simulink library "miniMUTT_rigid_Aero_Lib"  (Simulink 8.4)
settings: Solver=ode45  StartTime=0.0  StopTime=10.0  RelTol=1e-3
values from neighbouring files (symbols this model uses):
  AC = miniMUTT_rigid_config    [UAV_config.m]    (also in UAV_modelconfig.mat = )
libraries: simulink x1
settings Model: Creator=kotik001  LastModifiedBy=pseiler

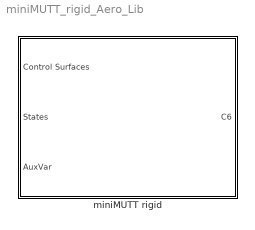
== system miniMUTT_rigid_Aero_Lib ==
  miniMUTT rigid : Subsystem

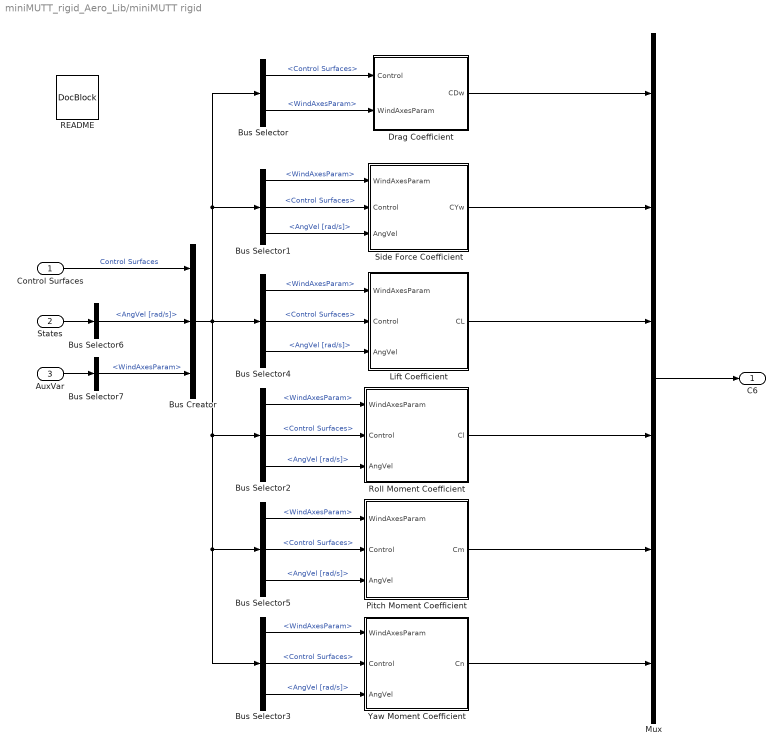
== system miniMUTT_rigid_Aero_Lib/miniMUTT rigid ==
  Control Surfaces : Inport
  States : Inport  Port=2
  AuxVar : Inport  Port=3
  Bus Creator : BusCreator  Inputs=3
  Bus Selector : BusSelector  OutputSignals=Control Surfaces,WindAxesParam
  Bus Selector{1..5} (5 alike) : BusSelector  OutputSignals=WindAxesParam,Control Surfaces,AngVel [rad/s]
  Bus Selector6 : BusSelector  OutputSignals=AngVel [rad/s]
  Bus Selector7 : BusSelector  OutputSignals=WindAxesParam
  Drag Coefficient : Subsystem
  Lift Coefficient : Subsystem
  Mux : Mux  Inputs=6
  Pitch Moment Coefficient : Subsystem
  README : simulink/Model-Wide Utilities/DocBlock  DocumentType=Text
  Roll Moment Coefficient : Subsystem
  Side Force Coefficient : Subsystem
  Yaw Moment Coefficient : Subsystem
  C6 : Outport
  wires:
  Bus Selector/2 -> Drag Coefficient/2(WindAxesParam)  "<WindAxesParam>"
  Bus Selector/1 -> Drag Coefficient/1(Control)  "<Control Surfaces>"
  Bus Selector5/3 -> Pitch Moment Coefficient/3(AngVel)  "<AngVel [rad/s]>"
  Bus Selector5/2 -> Pitch Moment Coefficient/2(Control)  "<Control Surfaces>"
  Bus Selector5/1 -> Pitch Moment Coefficient/1(WindAxesParam)  "<WindAxesParam>"
  Bus Selector4/3 -> Lift Coefficient/3(AngVel)  "<AngVel [rad/s]>"
  Bus Selector4/2 -> Lift Coefficient/2(Control)  "<Control Surfaces>"
  Bus Selector4/1 -> Lift Coefficient/1(WindAxesParam)  "<WindAxesParam>"
  Bus Selector3/3 -> Yaw Moment Coefficient/3(AngVel)  "<AngVel [rad/s]>"
  Bus Selector3/2 -> Yaw Moment Coefficient/2(Control)  "<Control Surfaces>"
  Bus Selector3/1 -> Yaw Moment Coefficient/1(WindAxesParam)  "<WindAxesParam>"
  Bus Selector2/3 -> Roll Moment Coefficient/3(AngVel)  "<AngVel [rad/s]>"
  Bus Selector2/2 -> Roll Moment Coefficient/2(Control)  "<Control Surfaces>"
  Bus Selector2/1 -> Roll Moment Coefficient/1(WindAxesParam)  "<WindAxesParam>"
  Bus Selector1/3 -> Side Force Coefficient/3(AngVel)  "<AngVel [rad/s]>"
  Bus Selector1/2 -> Side Force Coefficient/2(Control)  "<Control Surfaces>"
  Bus Selector1/1 -> Side Force Coefficient/1(WindAxesParam)  "<WindAxesParam>"
  Bus Creator/1 -> Bus Selector1/1, Bus Selector/1, Bus Selector4/1, Bus Selector5/1, Bus Selector3/1, Bus Selector2/1
  Mux/1 -> C6/1
  Yaw Moment Coefficient/1(Cn) -> Mux/6
  Pitch Moment Coefficient/1(Cm) -> Mux/5
  Roll Moment Coefficient/1(Cl) -> Mux/4
  Side Force Coefficient/1(CYw) -> Mux/2
  Drag Coefficient/1(CDw) -> Mux/1
  States/1 -> Bus Selector6/1
  Bus Selector6/1 -> Bus Creator/2  "<AngVel [rad/s]>"
  Lift Coefficient/1(CL) -> Mux/3
  AuxVar/1 -> Bus Selector7/1
  Bus Selector7/1 -> Bus Creator/3  "<WindAxesParam>"
  Control Surfaces/1 -> Bus Creator/1  "Control Surfaces"

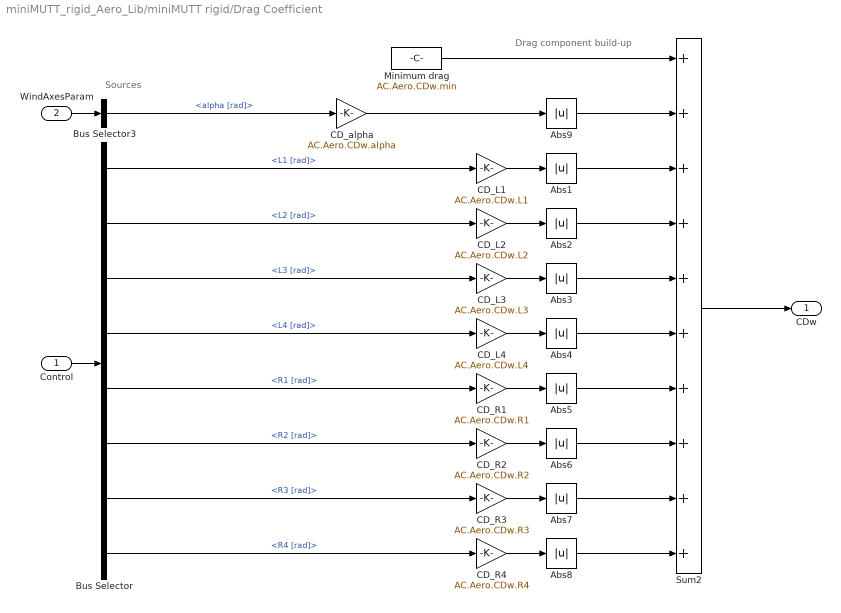
== system miniMUTT_rigid_Aero_Lib/miniMUTT rigid/Drag Coefficient ==
  note: Sources
  note: Drag component build-up
  Control : Inport
  WindAxesParam : Inport  Port=2
  Abs{1..9} (9 alike) : Abs  SaturateOnIntegerOverflow=on
  Bus Selector : BusSelector  OutputSignals=L1 [rad],L2 [rad],L3 [rad],L4 [rad],R1 [rad],R2 [rad],R3 [rad],R4 [rad]
  Bus Selector3 : BusSelector  OutputSignals=alpha [rad]
  CD_L1 : Gain  Gain=AC.Aero.CDw.L1  SaturateOnIntegerOverflow=on  OutDataTypeStr=Inherit: Same as input  ParamDataTypeStr=Inherit: Same as input
  CD_L2 : Gain  Gain=AC.Aero.CDw.L2  SaturateOnIntegerOverflow=on  OutDataTypeStr=Inherit: Same as input  ParamDataTypeStr=Inherit: Same as input
  CD_L3 : Gain  Gain=AC.Aero.CDw.L3  SaturateOnIntegerOverflow=on  OutDataTypeStr=Inherit: Same as input  ParamDataTypeStr=Inherit: Same as input
  CD_L4 : Gain  Gain=AC.Aero.CDw.L4  SaturateOnIntegerOverflow=on  OutDataTypeStr=Inherit: Same as input  ParamDataTypeStr=Inherit: Same as input
  CD_R1 : Gain  Gain=AC.Aero.CDw.R1  SaturateOnIntegerOverflow=on  OutDataTypeStr=Inherit: Same as input  ParamDataTypeStr=Inherit: Same as input
  CD_R2 : Gain  Gain=AC.Aero.CDw.R2  SaturateOnIntegerOverflow=on  OutDataTypeStr=Inherit: Same as input  ParamDataTypeStr=Inherit: Same as input
  CD_R3 : Gain  Gain=AC.Aero.CDw.R3  SaturateOnIntegerOverflow=on  OutDataTypeStr=Inherit: Same as input  ParamDataTypeStr=Inherit: Same as input
  CD_R4 : Gain  Gain=AC.Aero.CDw.R4  SaturateOnIntegerOverflow=on  OutDataTypeStr=Inherit: Same as input  ParamDataTypeStr=Inherit: Same as input
  CD_alpha : Gain  Gain=AC.Aero.CDw.alpha  SaturateOnIntegerOverflow=on  OutDataTypeStr=Inherit: Same as input  ParamDataTypeStr=Inherit: Same as input
  Minimum drag : Constant  Value=AC.Aero.CDw.min
  Sum2 : Sum  Inputs=++++++++++  SaturateOnIntegerOverflow=on  InputSameDT=on  OutDataTypeStr=Inherit: Same as first input
  CDw : Outport
  wires:
  WindAxesParam/1 -> Bus Selector3/1
  Bus Selector3/1 -> CD_alpha/1  "<alpha [rad]>"
  Bus Selector/7 -> CD_R3/1  "<R3 [rad]>"
  CD_R3/1 -> Abs7/1
  CD_R4/1 -> Abs8/1
  Abs8/1 -> Sum2/10
  Abs7/1 -> Sum2/9
  Bus Selector/8 -> CD_R4/1  "<R4 [rad]>"
  Bus Selector/5 -> CD_R1/1  "<R1 [rad]>"
  Bus Selector/1 -> CD_L1/1  "<L1 [rad]>"
  Bus Selector/2 -> CD_L2/1  "<L2 [rad]>"
  Control/1 -> Bus Selector/1
  Minimum drag/1 -> Sum2/1
  CD_R1/1 -> Abs5/1
  CD_L1/1 -> Abs1/1
  CD_L4/1 -> Abs4/1
  CD_L2/1 -> Abs2/1
  Sum2/1 -> CDw/1
  Abs1/1 -> Sum2/3
  Abs2/1 -> Sum2/4
  Bus Selector/4 -> CD_L4/1  "<L4 [rad]>"
  Abs4/1 -> Sum2/6
  CD_L3/1 -> Abs3/1
  Abs3/1 -> Sum2/5
  Bus Selector/3 -> CD_L3/1  "<L3 [rad]>"
  CD_R2/1 -> Abs6/1
  Abs6/1 -> Sum2/8
  Abs5/1 -> Sum2/7
  Bus Selector/6 -> CD_R2/1  "<R2 [rad]>"
  Abs9/1 -> Sum2/2
  CD_alpha/1 -> Abs9/1

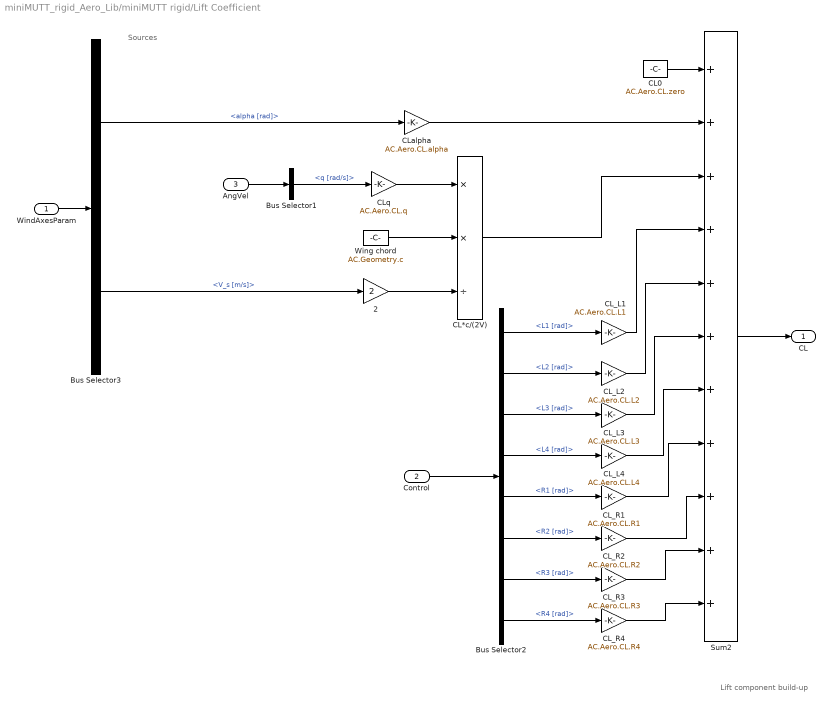
== system miniMUTT_rigid_Aero_Lib/miniMUTT rigid/Lift Coefficient ==
  note: Sources
  note: Lift component build-up
  WindAxesParam : Inport
  Control : Inport  Port=2
  AngVel : Inport  Port=3
  2 : Gain  Gain=2  SaturateOnIntegerOverflow=on  OutDataTypeStr=Inherit: Same as input  ParamDataTypeStr=Inherit: Same as input
  Bus Selector1 : BusSelector  OutputSignals=q [rad/s]
  Bus Selector2 : BusSelector  OutputSignals=L1 [rad],L2 [rad],L3 [rad],L4 [rad],R1 [rad],R2 [rad],R3 [rad],R4 [rad]
  Bus Selector3 : BusSelector  OutputSignals=alpha [rad],V_s [m/s]
  CL*c/(2V) : Product  Inputs=**/  SaturateOnIntegerOverflow=on  InputSameDT=on  OutDataTypeStr=Inherit: Same as first input
  CL0 : Constant  Value=AC.Aero.CL.zero
  CL_L1 : Gain  Gain=AC.Aero.CL.L1  SaturateOnIntegerOverflow=on  OutDataTypeStr=Inherit: Same as input  ParamDataTypeStr=Inherit: Same as input
  CL_L2 : Gain  Gain=AC.Aero.CL.L2  SaturateOnIntegerOverflow=on  OutDataTypeStr=Inherit: Same as input  ParamDataTypeStr=Inherit: Same as input
  CL_L3 : Gain  Gain=AC.Aero.CL.L3  SaturateOnIntegerOverflow=on  OutDataTypeStr=Inherit: Same as input  ParamDataTypeStr=Inherit: Same as input
  CL_L4 : Gain  Gain=AC.Aero.CL.L4  SaturateOnIntegerOverflow=on  OutDataTypeStr=Inherit: Same as input  ParamDataTypeStr=Inherit: Same as input
  CL_R1 : Gain  Gain=AC.Aero.CL.R1  SaturateOnIntegerOverflow=on  OutDataTypeStr=Inherit: Same as input  ParamDataTypeStr=Inherit: Same as input
  CL_R2 : Gain  Gain=AC.Aero.CL.R2  SaturateOnIntegerOverflow=on  OutDataTypeStr=Inherit: Same as input  ParamDataTypeStr=Inherit: Same as input
  CL_R3 : Gain  Gain=AC.Aero.CL.R3  SaturateOnIntegerOverflow=on  OutDataTypeStr=Inherit: Same as input  ParamDataTypeStr=Inherit: Same as input
  CL_R4 : Gain  Gain=AC.Aero.CL.R4  SaturateOnIntegerOverflow=on  OutDataTypeStr=Inherit: Same as input  ParamDataTypeStr=Inherit: Same as input
  CLalpha : Gain  Gain=AC.Aero.CL.alpha  SaturateOnIntegerOverflow=on  OutDataTypeStr=Inherit: Same as input  ParamDataTypeStr=Inherit: Same as input
  CLq : Gain  Gain=AC.Aero.CL.q  SaturateOnIntegerOverflow=on  OutDataTypeStr=Inherit: Same as input  ParamDataTypeStr=Inherit: Same as input
  Sum2 : Sum  Inputs=+++++++++++  SaturateOnIntegerOverflow=on  InputSameDT=on  OutDataTypeStr=Inherit: Same as first input
  Wing chord : Constant  Value=AC.Geometry.c
  CL : Outport
  wires:
  CL_R4/1 -> Sum2/11
  CL_R3/1 -> Sum2/10
  CL_R2/1 -> Sum2/9
  Bus Selector2/6 -> CL_R2/1  "<R2 [rad]>"
  Bus Selector2/7 -> CL_R3/1  "<R3 [rad]>"
  Bus Selector2/8 -> CL_R4/1  "<R4 [rad]>"
  WindAxesParam/1 -> Bus Selector3/1
  CL0/1 -> Sum2/1
  CLalpha/1 -> Sum2/2
  Sum2/1 -> CL/1
  Bus Selector3/1 -> CLalpha/1  "<alpha [rad]>"
  Control/1 -> Bus Selector2/1
  Bus Selector2/1 -> CL_L1/1  "<L1 [rad]>"
  2/1 -> CL*c/(2V)/3
  Wing chord/1 -> CL*c/(2V)/2
  CLq/1 -> CL*c/(2V)/1
  AngVel/1 -> Bus Selector1/1
  Bus Selector1/1 -> CLq/1  "<q [rad/s]>"
  Bus Selector3/2 -> 2/1  "<V_s [m/s]>"
  CL*c/(2V)/1 -> Sum2/3
  CL_L1/1 -> Sum2/4
  Bus Selector2/2 -> CL_L2/1  "<L2 [rad]>"
  Bus Selector2/3 -> CL_L3/1  "<L3 [rad]>"
  Bus Selector2/4 -> CL_L4/1  "<L4 [rad]>"
  Bus Selector2/5 -> CL_R1/1  "<R1 [rad]>"
  CL_L4/1 -> Sum2/7
  CL_R1/1 -> Sum2/8
  CL_L3/1 -> Sum2/6
  CL_L2/1 -> Sum2/5

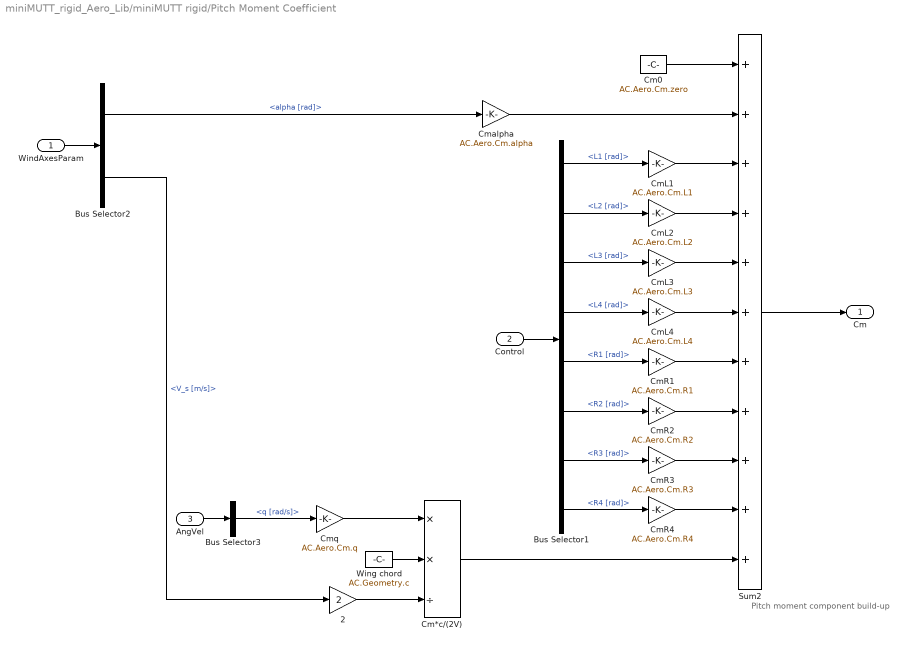
== system miniMUTT_rigid_Aero_Lib/miniMUTT rigid/Pitch Moment Coefficient ==
  note: Pitch moment component build-up
  WindAxesParam : Inport
  Control : Inport  Port=2
  AngVel : Inport  Port=3
  2 : Gain  Gain=2  SaturateOnIntegerOverflow=on  OutDataTypeStr=Inherit: Same as input  ParamDataTypeStr=Inherit: Same as input
  Bus Selector1 : BusSelector  OutputSignals=L1 [rad],L2 [rad],L3 [rad],L4 [rad],R1 [rad],R2 [rad],R3 [rad],R4 [rad]
  Bus Selector2 : BusSelector  OutputSignals=alpha [rad],V_s [m/s]
  Bus Selector3 : BusSelector  OutputSignals=q [rad/s]
  Cm*c/(2V) : Product  Inputs=**/  SaturateOnIntegerOverflow=on  RndMeth=Zero  InputSameDT=on  OutDataTypeStr=Inherit: Same as first input
  Cm0 : Constant  Value=AC.Aero.Cm.zero
  CmL1 : Gain  Gain=AC.Aero.Cm.L1  SaturateOnIntegerOverflow=on  OutDataTypeStr=Inherit: Same as input  ParamDataTypeStr=Inherit: Same as input
  CmL2 : Gain  Gain=AC.Aero.Cm.L2  SaturateOnIntegerOverflow=on  OutDataTypeStr=Inherit: Same as input  ParamDataTypeStr=Inherit: Same as input
  CmL3 : Gain  Gain=AC.Aero.Cm.L3  SaturateOnIntegerOverflow=on  OutDataTypeStr=Inherit: Same as input  ParamDataTypeStr=Inherit: Same as input
  CmL4 : Gain  Gain=AC.Aero.Cm.L4  SaturateOnIntegerOverflow=on  OutDataTypeStr=Inherit: Same as input  ParamDataTypeStr=Inherit: Same as input
  CmR1 : Gain  Gain=AC.Aero.Cm.R1  SaturateOnIntegerOverflow=on  OutDataTypeStr=Inherit: Same as input  ParamDataTypeStr=Inherit: Same as input
  CmR2 : Gain  Gain=AC.Aero.Cm.R2  SaturateOnIntegerOverflow=on  OutDataTypeStr=Inherit: Same as input  ParamDataTypeStr=Inherit: Same as input
  CmR3 : Gain  Gain=AC.Aero.Cm.R3  SaturateOnIntegerOverflow=on  OutDataTypeStr=Inherit: Same as input  ParamDataTypeStr=Inherit: Same as input
  CmR4 : Gain  Gain=AC.Aero.Cm.R4  SaturateOnIntegerOverflow=on  OutDataTypeStr=Inherit: Same as input  ParamDataTypeStr=Inherit: Same as input
  Cmalpha : Gain  Gain=AC.Aero.Cm.alpha  SaturateOnIntegerOverflow=on  OutDataTypeStr=Inherit: Same as input  ParamDataTypeStr=Inherit: Same as input
  Cmq : Gain  Gain=AC.Aero.Cm.q  SaturateOnIntegerOverflow=on  OutDataTypeStr=Inherit: Same as input  ParamDataTypeStr=Inherit: Same as input
  Sum2 : Sum  Inputs=+++++++++++  SaturateOnIntegerOverflow=on  InputSameDT=on  OutDataTypeStr=Inherit: Same as first input
  Wing chord : Constant  Value=AC.Geometry.c
  Cm : Outport
  wires:
  CmR2/1 -> Sum2/8
  CmR3/1 -> Sum2/9
  CmR4/1 -> Sum2/10
  Bus Selector1/6 -> CmR2/1  "<R2 [rad]>"
  Bus Selector1/7 -> CmR3/1  "<R3 [rad]>"
  Bus Selector1/8 -> CmR4/1  "<R4 [rad]>"
  Cm*c/(2V)/1 -> Sum2/11
  WindAxesParam/1 -> Bus Selector2/1
  Control/1 -> Bus Selector1/1
  AngVel/1 -> Bus Selector3/1
  2/1 -> Cm*c/(2V)/3
  Wing chord/1 -> Cm*c/(2V)/2
  Cmq/1 -> Cm*c/(2V)/1
  Cm0/1 -> Sum2/1
  Cmalpha/1 -> Sum2/2
  Sum2/1 -> Cm/1
  Bus Selector3/1 -> Cmq/1  "<q [rad/s]>"
  Bus Selector2/1 -> Cmalpha/1  "<alpha [rad]>"
  Bus Selector2/2 -> 2/1  "<V_s [m/s]>"
  CmL1/1 -> Sum2/3
  CmL2/1 -> Sum2/4
  CmL3/1 -> Sum2/5
  CmL4/1 -> Sum2/6
  CmR1/1 -> Sum2/7
  Bus Selector1/1 -> CmL1/1  "<L1 [rad]>"
  Bus Selector1/2 -> CmL2/1  "<L2 [rad]>"
  Bus Selector1/3 -> CmL3/1  "<L3 [rad]>"
  Bus Selector1/4 -> CmL4/1  "<L4 [rad]>"
  Bus Selector1/5 -> CmR1/1  "<R1 [rad]>"

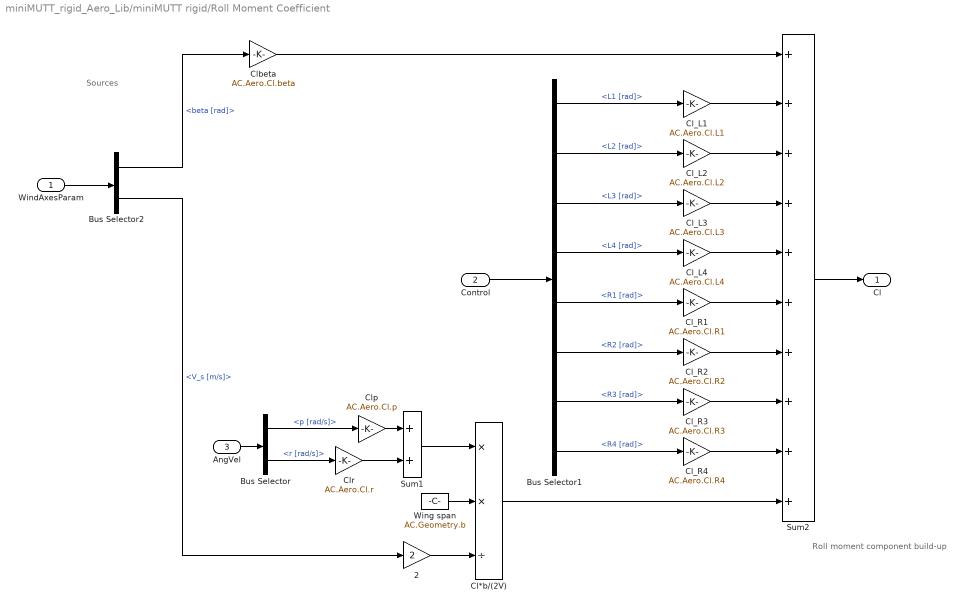
== system miniMUTT_rigid_Aero_Lib/miniMUTT rigid/Roll Moment Coefficient ==
  note: Sources
  note: Roll moment component build-up
  WindAxesParam : Inport
  Control : Inport  Port=2
  AngVel : Inport  Port=3
  2 : Gain  Gain=2  SaturateOnIntegerOverflow=on  OutDataTypeStr=Inherit: Same as input  ParamDataTypeStr=Inherit: Same as input
  Bus Selector : BusSelector  OutputSignals=p [rad/s],r [rad/s]
  Bus Selector1 : BusSelector  OutputSignals=L1 [rad],L2 [rad],L3 [rad],L4 [rad],R1 [rad],R2 [rad],R3 [rad],R4 [rad]
  Bus Selector2 : BusSelector  OutputSignals=beta [rad],V_s [m/s]
  Cl*b/(2V) : Product  Inputs=**/  SaturateOnIntegerOverflow=on  RndMeth=Zero  InputSameDT=on  OutDataTypeStr=Inherit: Same as first input
  Cl_L1 : Gain  Gain=AC.Aero.Cl.L1  SaturateOnIntegerOverflow=on  OutDataTypeStr=Inherit: Same as input  ParamDataTypeStr=Inherit: Same as input
  Cl_L2 : Gain  Gain=AC.Aero.Cl.L2  SaturateOnIntegerOverflow=on  OutDataTypeStr=Inherit: Same as input  ParamDataTypeStr=Inherit: Same as input
  Cl_L3 : Gain  Gain=AC.Aero.Cl.L3  SaturateOnIntegerOverflow=on  OutDataTypeStr=Inherit: Same as input  ParamDataTypeStr=Inherit: Same as input
  Cl_L4 : Gain  Gain=AC.Aero.Cl.L4  SaturateOnIntegerOverflow=on  OutDataTypeStr=Inherit: Same as input  ParamDataTypeStr=Inherit: Same as input
  Cl_R1 : Gain  Gain=AC.Aero.Cl.R1  SaturateOnIntegerOverflow=on  OutDataTypeStr=Inherit: Same as input  ParamDataTypeStr=Inherit: Same as input
  Cl_R2 : Gain  Gain=AC.Aero.Cl.R2  SaturateOnIntegerOverflow=on  OutDataTypeStr=Inherit: Same as input  ParamDataTypeStr=Inherit: Same as input
  Cl_R3 : Gain  Gain=AC.Aero.Cl.R3  SaturateOnIntegerOverflow=on  OutDataTypeStr=Inherit: Same as input  ParamDataTypeStr=Inherit: Same as input
  Cl_R4 : Gain  Gain=AC.Aero.Cl.R4  SaturateOnIntegerOverflow=on  OutDataTypeStr=Inherit: Same as input  ParamDataTypeStr=Inherit: Same as input
  Clbeta : Gain  Gain=AC.Aero.Cl.beta  SaturateOnIntegerOverflow=on  OutDataTypeStr=Inherit: Same as input  ParamDataTypeStr=Inherit: Same as input
  Clp : Gain  Gain=AC.Aero.Cl.p  SaturateOnIntegerOverflow=on  OutDataTypeStr=Inherit: Same as input  ParamDataTypeStr=Inherit: Same as input
  Clr : Gain  Gain=AC.Aero.Cl.r  SaturateOnIntegerOverflow=on  OutDataTypeStr=Inherit: Same as input  ParamDataTypeStr=Inherit: Same as input
  Sum1 : Sum  SaturateOnIntegerOverflow=on  InputSameDT=on  OutDataTypeStr=Inherit: Same as first input
  Sum2 : Sum  Inputs=++++++++++  SaturateOnIntegerOverflow=on  InputSameDT=on  OutDataTypeStr=Inherit: Same as first input
  Wing span : Constant  Value=AC.Geometry.b
  Cl : Outport
  wires:
  Control/1 -> Bus Selector1/1
  Bus Selector1/6 -> Cl_R2/1  "<R2 [rad]>"
  Cl_R2/1 -> Sum2/7
  Bus Selector1/7 -> Cl_R3/1  "<R3 [rad]>"
  Bus Selector1/8 -> Cl_R4/1  "<R4 [rad]>"
  Cl_R3/1 -> Sum2/8
  Cl_R4/1 -> Sum2/9
  Cl*b/(2V)/1 -> Sum2/10
  Clp/1 -> Sum1/1
  Clr/1 -> Sum1/2
  Sum1/1 -> Cl*b/(2V)/1
  Wing span/1 -> Cl*b/(2V)/2
  2/1 -> Cl*b/(2V)/3
  WindAxesParam/1 -> Bus Selector2/1
  AngVel/1 -> Bus Selector/1
  Clbeta/1 -> Sum2/1
  Sum2/1 -> Cl/1
  Bus Selector/1 -> Clp/1  "<p [rad/s]>"
  Bus Selector/2 -> Clr/1  "<r [rad/s]>"
  Bus Selector1/1 -> Cl_L1/1  "<L1 [rad]>"
  Bus Selector2/1 -> Clbeta/1  "<beta [rad]>"
  Bus Selector2/2 -> 2/1  "<V_s [m/s]>"
  Cl_L1/1 -> Sum2/2
  Cl_L2/1 -> Sum2/3
  Bus Selector1/2 -> Cl_L2/1  "<L2 [rad]>"
  Bus Selector1/3 -> Cl_L3/1  "<L3 [rad]>"
  Cl_L3/1 -> Sum2/4
  Bus Selector1/4 -> Cl_L4/1  "<L4 [rad]>"
  Bus Selector1/5 -> Cl_R1/1  "<R1 [rad]>"
  Cl_L4/1 -> Sum2/5
  Cl_R1/1 -> Sum2/6

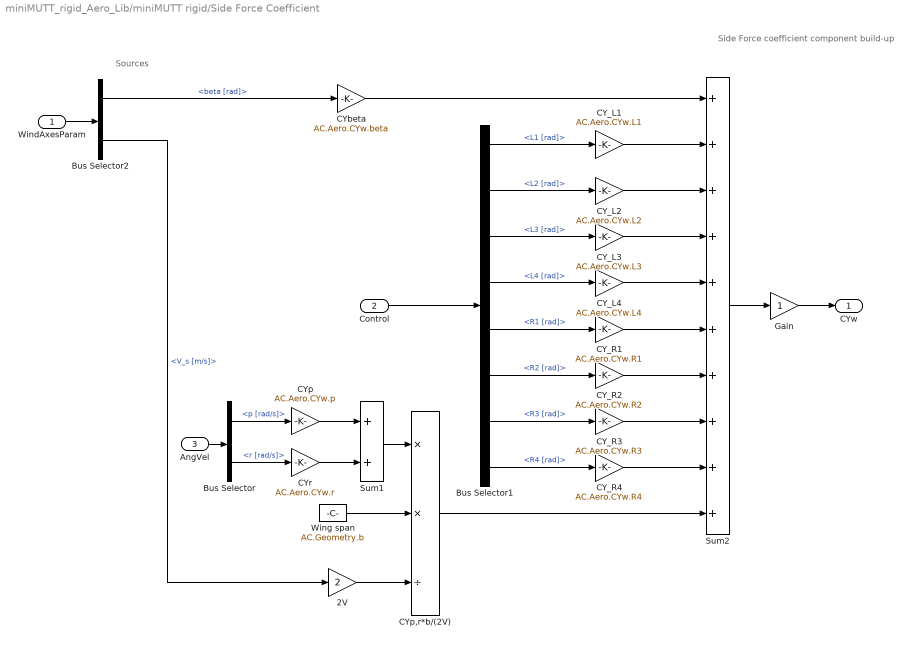
== system miniMUTT_rigid_Aero_Lib/miniMUTT rigid/Side Force Coefficient ==
  note: Sources
  note: Side Force coefficient component build-up
  WindAxesParam : Inport
  Control : Inport  Port=2
  AngVel : Inport  Port=3
  2V : Gain  Gain=2  SaturateOnIntegerOverflow=on  OutDataTypeStr=Inherit: Same as input  ParamDataTypeStr=Inherit: Same as input
  Bus Selector : BusSelector  OutputSignals=p [rad/s],r [rad/s]
  Bus Selector1 : BusSelector  OutputSignals=L1 [rad],L2 [rad],L3 [rad],L4 [rad],R1 [rad],R2 [rad],R3 [rad],R4 [rad]
  Bus Selector2 : BusSelector  OutputSignals=beta [rad],V_s [m/s]
  CY_L1 : Gain  Gain=AC.Aero.CYw.L1  SaturateOnIntegerOverflow=on  OutDataTypeStr=Inherit: Same as input  ParamDataTypeStr=Inherit: Same as input
  CY_L2 : Gain  Gain=AC.Aero.CYw.L2  SaturateOnIntegerOverflow=on  OutDataTypeStr=Inherit: Same as input  ParamDataTypeStr=Inherit: Same as input
  CY_L3 : Gain  Gain=AC.Aero.CYw.L3  SaturateOnIntegerOverflow=on  OutDataTypeStr=Inherit: Same as input  ParamDataTypeStr=Inherit: Same as input
  CY_L4 : Gain  Gain=AC.Aero.CYw.L4  SaturateOnIntegerOverflow=on  OutDataTypeStr=Inherit: Same as input  ParamDataTypeStr=Inherit: Same as input
  CY_R1 : Gain  Gain=AC.Aero.CYw.R1  SaturateOnIntegerOverflow=on  OutDataTypeStr=Inherit: Same as input  ParamDataTypeStr=Inherit: Same as input
  CY_R2 : Gain  Gain=AC.Aero.CYw.R2  SaturateOnIntegerOverflow=on  OutDataTypeStr=Inherit: Same as input  ParamDataTypeStr=Inherit: Same as input
  CY_R3 : Gain  Gain=AC.Aero.CYw.R3  SaturateOnIntegerOverflow=on  OutDataTypeStr=Inherit: Same as input  ParamDataTypeStr=Inherit: Same as input
  CY_R4 : Gain  Gain=AC.Aero.CYw.R4  SaturateOnIntegerOverflow=on  OutDataTypeStr=Inherit: Same as input  ParamDataTypeStr=Inherit: Same as input
  CYbeta : Gain  Gain=AC.Aero.CYw.beta  SaturateOnIntegerOverflow=on  OutDataTypeStr=Inherit: Same as input  ParamDataTypeStr=Inherit: Same as input
  CYp : Gain  Gain=AC.Aero.CYw.p  SaturateOnIntegerOverflow=on  OutDataTypeStr=Inherit: Same as input  ParamDataTypeStr=Inherit: Same as input
  CYp,r*b/(2V) : Product  Inputs=**/  SaturateOnIntegerOverflow=on  RndMeth=Zero  InputSameDT=on  OutDataTypeStr=Inherit: Same as first input
  CYr : Gain  Gain=AC.Aero.CYw.r  SaturateOnIntegerOverflow=on  OutDataTypeStr=Inherit: Same as input  ParamDataTypeStr=Inherit: Same as input
  Gain : Gain
  Sum1 : Sum  SaturateOnIntegerOverflow=on  InputSameDT=on  OutDataTypeStr=Inherit: Same as first input
  Sum2 : Sum  Inputs=++++++++++  SaturateOnIntegerOverflow=on  InputSameDT=on  OutDataTypeStr=Inherit: Same as first input
  Wing span : Constant  Value=AC.Geometry.b
  CYw : Outport
  wires:
  CY_R4/1 -> Sum2/9
  CY_R3/1 -> Sum2/8
  Bus Selector1/8 -> CY_R4/1  "<R4 [rad]>"
  Bus Selector1/7 -> CY_R3/1  "<R3 [rad]>"
  CY_R2/1 -> Sum2/7
  CY_R1/1 -> Sum2/6
  CY_L4/1 -> Sum2/5
  Bus Selector1/4 -> CY_L4/1  "<L4 [rad]>"
  Bus Selector1/6 -> CY_R2/1  "<R2 [rad]>"
  Bus Selector1/5 -> CY_R1/1  "<R1 [rad]>"
  CYp,r*b/(2V)/1 -> Sum2/10
  CYp/1 -> Sum1/1
  CYr/1 -> Sum1/2
  Sum1/1 -> CYp,r*b/(2V)/1
  Wing span/1 -> CYp,r*b/(2V)/2
  2V/1 -> CYp,r*b/(2V)/3
  WindAxesParam/1 -> Bus Selector2/1
  Bus Selector/1 -> CYp/1  "<p [rad/s]>"
  CYbeta/1 -> Sum2/1
  CY_L1/1 -> Sum2/2
  Sum2/1 -> Gain/1
  AngVel/1 -> Bus Selector/1
  Bus Selector/2 -> CYr/1  "<r [rad/s]>"
  Control/1 -> Bus Selector1/1
  Bus Selector1/1 -> CY_L1/1  "<L1 [rad]>"
  Bus Selector1/3 -> CY_L3/1  "<L3 [rad]>"
  Bus Selector2/2 -> 2V/1  "<V_s [m/s]>"
  Bus Selector2/1 -> CYbeta/1  "<beta [rad]>"
  Gain/1 -> CYw/1
  CY_L3/1 -> Sum2/4
  Bus Selector1/2 -> CY_L2/1  "<L2 [rad]>"
  CY_L2/1 -> Sum2/3

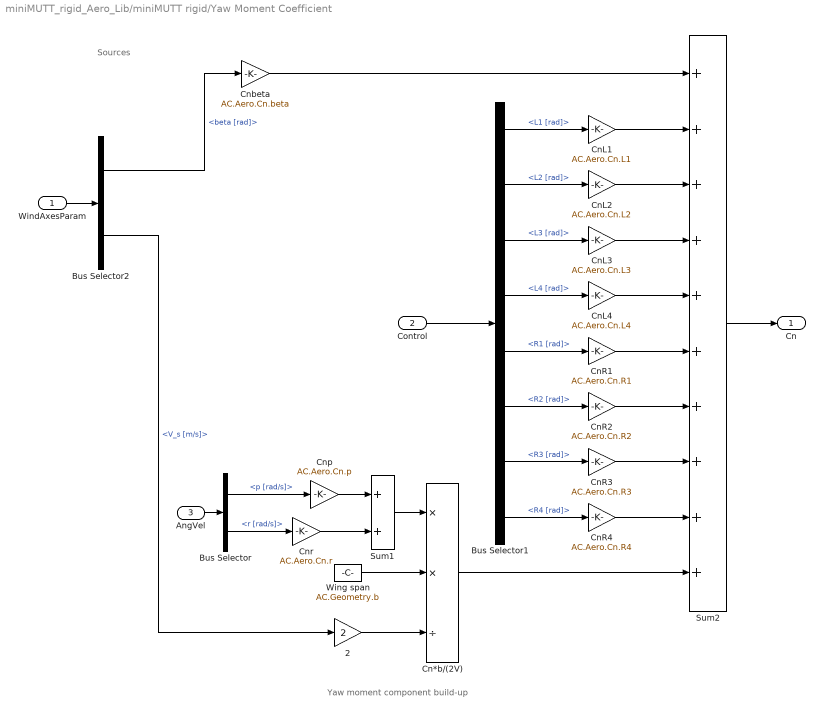
== system miniMUTT_rigid_Aero_Lib/miniMUTT rigid/Yaw Moment Coefficient ==
  note: Yaw moment component build-up
  note: Sources
  WindAxesParam : Inport
  Control : Inport  Port=2
  AngVel : Inport  Port=3
  2 : Gain  Gain=2  SaturateOnIntegerOverflow=on  OutDataTypeStr=Inherit: Same as input  ParamDataTypeStr=Inherit: Same as input
  Bus Selector : BusSelector  OutputSignals=p [rad/s],r [rad/s]
  Bus Selector1 : BusSelector  OutputSignals=L1 [rad],L2 [rad],L3 [rad],L4 [rad],R1 [rad],R2 [rad],R3 [rad],R4 [rad]
  Bus Selector2 : BusSelector  OutputSignals=beta [rad],V_s [m/s]
  Cn*b/(2V) : Product  Inputs=**/  SaturateOnIntegerOverflow=on  RndMeth=Zero  InputSameDT=on  OutDataTypeStr=Inherit: Same as first input
  CnL1 : Gain  Gain=AC.Aero.Cn.L1  SaturateOnIntegerOverflow=on  OutDataTypeStr=Inherit: Same as input  ParamDataTypeStr=Inherit: Same as input
  CnL2 : Gain  Gain=AC.Aero.Cn.L2  SaturateOnIntegerOverflow=on  OutDataTypeStr=Inherit: Same as input  ParamDataTypeStr=Inherit: Same as input
  CnL3 : Gain  Gain=AC.Aero.Cn.L3  SaturateOnIntegerOverflow=on  OutDataTypeStr=Inherit: Same as input  ParamDataTypeStr=Inherit: Same as input
  CnL4 : Gain  Gain=AC.Aero.Cn.L4  SaturateOnIntegerOverflow=on  OutDataTypeStr=Inherit: Same as input  ParamDataTypeStr=Inherit: Same as input
  CnR1 : Gain  Gain=AC.Aero.Cn.R1  SaturateOnIntegerOverflow=on  OutDataTypeStr=Inherit: Same as input  ParamDataTypeStr=Inherit: Same as input
  CnR2 : Gain  Gain=AC.Aero.Cn.R2  SaturateOnIntegerOverflow=on  OutDataTypeStr=Inherit: Same as input  ParamDataTypeStr=Inherit: Same as input
  CnR3 : Gain  Gain=AC.Aero.Cn.R3  SaturateOnIntegerOverflow=on  OutDataTypeStr=Inherit: Same as input  ParamDataTypeStr=Inherit: Same as input
  CnR4 : Gain  Gain=AC.Aero.Cn.R4  SaturateOnIntegerOverflow=on  OutDataTypeStr=Inherit: Same as input  ParamDataTypeStr=Inherit: Same as input
  Cnbeta : Gain  Gain=AC.Aero.Cn.beta  SaturateOnIntegerOverflow=on  OutDataTypeStr=Inherit: Same as input  ParamDataTypeStr=Inherit: Same as input
  Cnp : Gain  Gain=AC.Aero.Cn.p  SaturateOnIntegerOverflow=on  OutDataTypeStr=Inherit: Same as input  ParamDataTypeStr=Inherit: Same as input
  Cnr : Gain  Gain=AC.Aero.Cn.r  SaturateOnIntegerOverflow=on  OutDataTypeStr=Inherit: Same as input  ParamDataTypeStr=Inherit: Same as input
  Sum1 : Sum  SaturateOnIntegerOverflow=on  InputSameDT=on  OutDataTypeStr=Inherit: Same as first input
  Sum2 : Sum  Inputs=++++++++++  SaturateOnIntegerOverflow=on  InputSameDT=on  OutDataTypeStr=Inherit: Same as first input
  Wing span : Constant  Value=AC.Geometry.b
  Cn : Outport
  wires:
  CnR2/1 -> Sum2/7
  CnR3/1 -> Sum2/8
  CnR4/1 -> Sum2/9
  Bus Selector1/6 -> CnR2/1  "<R2 [rad]>"
  Bus Selector1/7 -> CnR3/1  "<R3 [rad]>"
  Bus Selector1/8 -> CnR4/1  "<R4 [rad]>"
  Cn*b/(2V)/1 -> Sum2/10
  Sum2/1 -> Cn/1
  Cnbeta/1 -> Sum2/1
  AngVel/1 -> Bus Selector/1
  WindAxesParam/1 -> Bus Selector2/1
  2/1 -> Cn*b/(2V)/3
  Wing span/1 -> Cn*b/(2V)/2
  Sum1/1 -> Cn*b/(2V)/1
  Cnr/1 -> Sum1/2
  Cnp/1 -> Sum1/1
  Bus Selector/1 -> Cnp/1  "<p [rad/s]>"
  Bus Selector/2 -> Cnr/1  "<r [rad/s]>"
  Control/1 -> Bus Selector1/1
  Bus Selector2/1 -> Cnbeta/1  "<beta [rad]>"
  Bus Selector2/2 -> 2/1  "<V_s [m/s]>"
  CnL3/1 -> Sum2/4
  CnL4/1 -> Sum2/5
  CnR1/1 -> Sum2/6
  Bus Selector1/1 -> CnL1/1  "<L1 [rad]>"
  Bus Selector1/2 -> CnL2/1  "<L2 [rad]>"
  Bus Selector1/3 -> CnL3/1  "<L3 [rad]>"
  Bus Selector1/4 -> CnL4/1  "<L4 [rad]>"
  Bus Selector1/5 -> CnR1/1  "<R1 [rad]>"
  CnL1/1 -> Sum2/2
  CnL2/1 -> Sum2/3
